simulink model "sl_basic"  (Simulink 6.6)
settings: Solver=FixedStepDiscrete  SolverMode=SingleTasking  StartTime=0.0  StopTime=10.0  RelTol=1e-3
settings Model: Creator=volgy  LastModifiedBy=vBuskirk
settings DebuggingCC: MultiTaskCondExecSysMsg=none
settings RTWCC: GenerateReport=on  LaunchReport=on  IncludeERTFirstTime=on

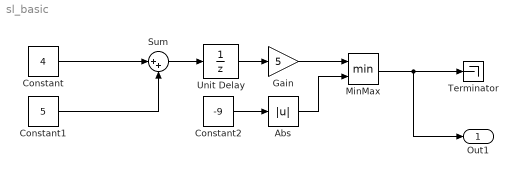
== system sl_basic ==
  Abs : Abs
  Constant : Constant  Value=4
  Constant1 : Constant  Value=5
  Constant2 : Constant  Value=-9
  Gain : Gain  Gain=5
  MinMax : MinMax  Inputs=2
  Sum : Sum  Inputs=|++
  Terminator : Terminator
  Unit Delay : UnitDelay
  Out1 : Outport
  wires:
  Constant/1 -> Sum/1
  Constant1/1 -> Sum/2
  Constant2/1 -> Abs/1
  Gain/1 -> MinMax/1
  Abs/1 -> MinMax/2
  Sum/1 -> Unit Delay/1
  Unit Delay/1 -> Gain/1
  MinMax/1 -> Out1/1, Terminator/1
